simulink model "sampleModel1417_5_sub_sub_sub"  (R2023a)
settings: Solver=VariableStepAuto  StartTime=0.0  StopTime=10.0  RelTol=1e-3
libraries: hdlsllib x6, simulink x3
settings Model: Creator=user1  LastModifiedBy=user1
settings OptimizationCC: BlockReduction=off  ConditionallyExecuteInputs=off

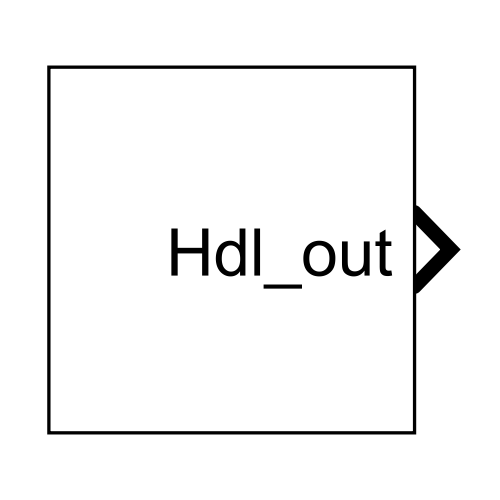
[thumbnail: Simulink's stored preview of the top-level diagram]
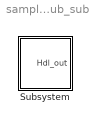
== system sampleModel1417_5_sub_sub_sub ==
  Subsystem : Subsystem

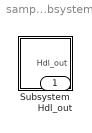
== system sampleModel1417_5_sub_sub_sub/Subsystem ==
  Subsystem : Subsystem
  Hdl_out : Outport  OutDataTypeStr=uint8

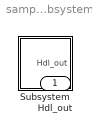
== system sampleModel1417_5_sub_sub_sub/Subsystem/Subsystem ==
  Subsystem : Subsystem
  Hdl_out : Outport  OutDataTypeStr=uint8

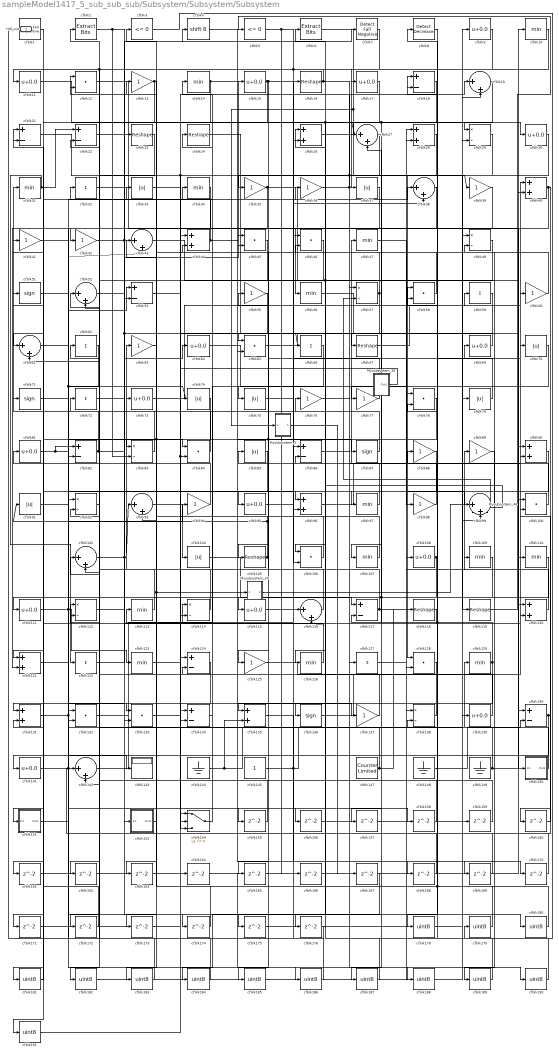
== system sampleModel1417_5_sub_sub_sub/Subsystem/Subsystem/Subsystem ==
  Mysubsystem_24 : Subsystem  TreatAsAtomicUnit=on  RTWFcnName=Mysubsystem_24
      settings: RTWFcnNameOpts=User specified  RTWFileNameOpts=Use function name
  Mysubsystem_35 : Subsystem  TreatAsAtomicUnit=on  RTWFcnName=Mysubsystem_35
      settings: RTWFcnNameOpts=User specified  RTWFileNameOpts=Use function name
  Mysubsystem_44 : Subsystem  TreatAsAtomicUnit=on  RTWFcnName=Mysubsystem_44
      settings: RTWFcnNameOpts=User specified  RTWFileNameOpts=Use function name
  Mysubsystem_5 : Subsystem  TreatAsAtomicUnit=on  RTWFcnName=Mysubsystem_5
      settings: RTWFcnNameOpts=User specified  RTWFileNameOpts=Use function name
  cfblk1 : hdlsllib/Logic and Bit Operations/Detect Fall Nonpositive  vinit=0  OutDataTypeStr=uint8
  cfblk{10,14,31,34,47,56,97,107,109..110,113,123,126,129} (14 alike) : MinMax  OutDataTypeStr=uint8
  cfblk{12,45..46,58,65,78,84,100,106,128,132..133} (12 alike) : DotProduct  OutDataTypeStr=uint8
  cfblk{19,27,38,43,52,61,93,99,102,116,142} (11 alike) : Sum  Inputs=|++  OutDataTypeStr=uint8
  cfblk{33,37,70,74..75,79,85,91,104} (9 alike) : Abs  OutDataTypeStr=uint8  SaturateOnIntegerOverflow=off
  cfblk{16,23..24,67,105,118..119} (7 alike) : Reshape
  cfblk{9,11,15,17,30,64,69,73,81,95,108,111,115,139,141} (15 alike) : Bias  Bias=0.0  SaturateOnIntegerOverflow=off
  cfblk{29,49,57,83,92,112,114,138} (8 alike) : Product  Inputs=*/  OutDataTypeStr=uint8  RndMeth=Zero  SaturateOnIntegerOverflow=on
  cfblk{18,21..22,53,82,86,117,124,134,140} (10 alike) : Sum  Inputs=+-  OutDataTypeStr=uint8
  cfblk{26,28,40,44,90,96,120..121,131,135} (10 alike) : Sum  OutDataTypeStr=uint8
  cfblk{32,59,62,66,72,122,127} (7 alike) : Sum  Inputs=+  OutDataTypeStr=uint8
  cfblk{13,35..36,39,41..42,55,60,63,76..77,88..89,94,98,125,137} (17 alike) : Gain  OutDataTypeStr=uint8
  cfblk{51,71,87,136} (4 alike) : Signum
  cfblk143 : Display
  cfblk144 : Ground
  cfblk145 : Constant  OutDataTypeStr=uint8  SampleTime=-1
  cfblk147 : hdlsllib/Sources/Counter Limited  uplimit=7  tsamp=-1
  cfblk148 : Ground
  cfblk149 : Ground
  cfblk150 : Subsystem
      settings: LibrarySourceBlock=|
      | hdlsllib/Ports &
      | Subsystems/Subsystem
  cfblk151 : Subsystem
      settings: LibrarySourceBlock=|
      | hdlsllib/Ports &
      | Subsystems/Subsystem
  cfblk153 : Subsystem
      settings: LibrarySourceBlock=|
      | hdlsllib/Ports &
      | Subsystems/Subsystem
  cfblk154 : Switch  OutDataTypeStr=uint8  SaturateOnIntegerOverflow=off  InputSameDT=off
  cfblk{155..176} (22 alike) : Delay  SampleTime=1
  cfblk{178..191} (14 alike) : DataTypeConversion  OutDataTypeStr=uint8  SaturateOnIntegerOverflow=off  RndMeth=Floor
  cfblk2 : simulink/Logic and Bit Operations/Extract Bits  bitsToExtract=Upper half  numBits=8  bitIdxRange=[0 7]  outScalingMode=Preserve fixed-point scaling
      settings: LibrarySourceBlock=|
      | hdlsllib/Logic and Bit
      | Operations/Extract Bits
  cfblk3 : hdlsllib/Logic and Bit Operations/Compare To Zero  relop=<=  OutDataTypeStr=uint8
  cfblk4 : ArithShift  BitShiftNumber=8
  cfblk5 : hdlsllib/Logic and Bit Operations/Compare To Zero  relop=<=  OutDataTypeStr=uint8
  cfblk6 : simulink/Logic and Bit Operations/Extract Bits  bitsToExtract=Upper half  numBits=8  bitIdxRange=[0 7]  outScalingMode=Preserve fixed-point scaling
      settings: LibrarySourceBlock=|
      | hdlsllib/Logic and Bit
      | Operations/Extract Bits
  cfblk7 : hdlsllib/Logic and Bit Operations/Detect Fall Negative  vinit=0  OutDataTypeStr=uint8
  cfblk8 : simulink/Logic and Bit Operations/Detect Decrease  vinit=0.0  OutDataTypeStr=uint8
      settings: LibrarySourceBlock=|
      | hdlsllib/Logic and Bit
      | Operations/Detect
      | Decrease
  Hdl_out : Outport  OutDataTypeStr=uint8
  wires:
  cfblk28/1 -> cfblk128/1
  cfblk81/1 -> cfblk53/1, cfblk82/1
  cfblk10/1 -> cfblk37/1
  cfblk69/1 -> cfblk65/1
  cfblk98/1 -> cfblk47/1
  cfblk125/1 -> cfblk40/1
  cfblk67/1 -> cfblk59/1
  cfblk114/1 -> cfblk63/1
  cfblk66/1 -> cfblk113/1
  cfblk119/1 -> cfblk5/1
  cfblk4/1 -> cfblk87/1
  cfblk84/1 -> cfblk32/1
  cfblk40/1 -> cfblk121/2, cfblk142/1
  cfblk142/1 -> cfblk114/1
  cfblk7/1 -> cfblk26/2, cfblk172/1, cfblk171/1
  cfblk16/1 -> cfblk11/1, cfblk168/1, cfblk39/1
  cfblk150/1(Out1) -> cfblk129/1
  cfblk102/1 -> cfblk45/2, cfblk93/1
  cfblk60/1 -> cfblk15/1
  cfblk65/1 -> cfblk67/1
  cfblk82/1 -> cfblk7/1, cfblk31/1
  cfblk1/1 -> cfblk61/1
  cfblk117/1 -> cfblk45/1, cfblk28/1
  cfblk87/1 -> cfblk21/1
  cfblk73/1 -> cfblk60/1
  cfblk120/1 -> cfblk89/1
  cfblk32/1 -> cfblk150/1(In1)
  cfblk12/1 -> cfblk56/1
  cfblk93/1 -> cfblk104/1
  cfblk39/1 -> cfblk96/1
  cfblk35/1 -> cfblk162/1, cfblk140/1
  cfblk139/1 -> cfblk73/1
  cfblk6/1 -> cfblk119/1, Mysubsystem_5/1(In1)
  cfblk106/1 -> cfblk71/1
  cfblk31/1 -> cfblk22/1, cfblk122/1
  cfblk26/1 -> cfblk30/1
  cfblk24/1 -> cfblk98/1
  cfblk53/1 -> cfblk44/1
  cfblk15/1 -> cfblk141/1, cfblk38/2, cfblk75/1
  cfblk148/1 -> cfblk140/2
  cfblk14/1 -> cfblk137/1, cfblk142/2
  cfblk9/1 -> cfblk17/1
  cfblk141/1 -> cfblk186/1, cfblk94/1
  cfblk21/1 -> cfblk57/1, cfblk114/2
  cfblk149/1 -> cfblk44/2, cfblk90/1
  cfblk43/1 -> cfblk100/1
  cfblk113/1 -> cfblk62/1
  cfblk104/1 -> cfblk117/1
  cfblk2/1 -> cfblk83/2, cfblk175/1, cfblk66/1
  cfblk34/1 -> cfblk132/2
  cfblk107/1 -> cfblk72/1
  cfblk116/1 -> cfblk2/1
  cfblk13/1 -> cfblk183/1, cfblk53/2
  cfblk37/1 -> cfblk83/1
  cfblk147/1 -> cfblk118/1, cfblk52/1
  cfblk96/1 -> cfblk40/2
  cfblk140/1 -> cfblk161/1, cfblk160/1
  cfblk115/1 -> cfblk16/1
  cfblk58/1 -> cfblk24/1
  cfblk56/1 -> cfblk110/1
  cfblk27/1 -> cfblk115/1
  cfblk62/1 -> cfblk82/2
  cfblk23/1 -> cfblk42/1
  cfblk132/1 -> cfblk86/1
  cfblk137/1 -> cfblk26/1
  cfblk5/1 -> cfblk166/1, cfblk78/1
  cfblk41/1 -> cfblk180/1
  cfblk74/1 -> cfblk121/1
  cfblk70/1 -> cfblk107/1
  cfblk128/1 -> cfblk124/2
  cfblk153/1(Out1) -> cfblk3/1
  cfblk49/1 -> cfblk116/2, cfblk102/2
  cfblk83/1 -> cfblk12/1
  cfblk61/1 -> cfblk84/1
  cfblk77/1 -> cfblk55/1
  cfblk78/1 -> cfblk165/1, cfblk191/1, cfblk163/1
  cfblk29/1 -> cfblk97/1
  cfblk75/1 -> cfblk70/1
  cfblk94/1 -> cfblk13/1
  cfblk17/1 -> cfblk106/1, cfblk133/1, Mysubsystem_24/1(In1)
  cfblk97/1 -> cfblk6/1
  cfblk112/1 -> cfblk120/2
  cfblk118/1 -> cfblk117/2
  cfblk127/1 -> cfblk109/1
  cfblk64/1 -> cfblk106/2
  cfblk42/1 -> cfblk4/1, cfblk153/1(In1)
  cfblk59/1 -> cfblk135/1
  cfblk111/1 -> cfblk133/2, cfblk123/1
  cfblk55/1 -> cfblk134/2
  cfblk144/1 -> cfblk135/2, cfblk9/1
  cfblk11/1 -> cfblk29/1
  cfblk72/1 -> cfblk96/2
  cfblk30/1 -> cfblk35/1
  cfblk126/1 -> cfblk51/1
  cfblk100/1 -> cfblk85/1
  cfblk47/1 -> cfblk99/1
  cfblk22/1 -> cfblk23/1
  cfblk86/1 -> cfblk90/2
  cfblk122/1 -> cfblk64/1
  cfblk63/1 -> cfblk33/1
  cfblk36/1 -> cfblk18/1, cfblk127/1
  cfblk79/1 -> cfblk58/1
  cfblk44/1 -> cfblk170/1, cfblk21/2
  cfblk131/1 -> cfblk43/2, cfblk143/1
  cfblk91/1 -> cfblk38/1
  cfblk108/1 -> cfblk18/2, cfblk187/1, cfblk136/1
  cfblk134/1 -> cfblk14/1
  cfblk129/1 -> cfblk131/1, cfblk88/1, cfblk27/2
  cfblk85/1 -> cfblk151/1(In1)
  cfblk95/1 -> cfblk69/1
  cfblk90/1 -> cfblk111/1
  cfblk124/1 -> cfblk154/2
  cfblk138/1 -> cfblk112/1
  cfblk105/1 -> cfblk125/1, cfblk81/1, cfblk91/1
  cfblk154/1 -> cfblk34/1
  cfblk151/1(Out1) -> cfblk138/2
  cfblk136/1 -> cfblk10/1
  cfblk123/1 -> cfblk19/1
  cfblk133/1 -> cfblk36/1
  cfblk19/1 -> cfblk105/1
  cfblk51/1 -> cfblk95/1, cfblk74/1
  cfblk18/1 -> cfblk77/1, cfblk27/1
  cfblk99/1 -> cfblk49/2
  cfblk145/1 -> cfblk29/2, cfblk116/1
  cfblk45/1 -> cfblk52/2
  cfblk57/1 -> cfblk12/2, cfblk65/2
  cfblk33/1 -> cfblk155/1
  cfblk155/1 -> cfblk102/1
  cfblk121/1 -> cfblk156/1
  cfblk156/1 -> cfblk128/2
  cfblk38/1 -> cfblk157/1
  cfblk157/1 -> cfblk19/2
  cfblk71/1 -> cfblk158/1
  cfblk158/1 -> cfblk61/2
  cfblk159/1 -> cfblk93/2
  cfblk160/1 -> cfblk100/2
  cfblk161/1 -> cfblk99/2
  cfblk162/1 -> cfblk22/2
  cfblk163/1 -> cfblk120/1
  cfblk165/1 -> cfblk28/2
  cfblk166/1 -> cfblk138/1
  cfblk168/1 -> cfblk112/2
  cfblk135/1 -> cfblk169/1
  cfblk169/1 -> cfblk132/1
  cfblk170/1 -> cfblk86/2
  cfblk171/1 -> cfblk124/1
  cfblk172/1 -> cfblk131/2
  cfblk109/1 -> cfblk173/1
  cfblk173/1 -> cfblk154/1
  cfblk52/1 -> cfblk174/1
  cfblk174/1 -> cfblk43/1
  cfblk175/1 -> cfblk49/1
  cfblk88/1 -> cfblk176/1
  cfblk176/1 -> cfblk1/1
  cfblk8/1 -> cfblk178/1
  cfblk178/1 -> cfblk139/1
  cfblk3/1 -> cfblk179/1
  cfblk179/1 -> cfblk8/1
  cfblk180/1 -> cfblk134/1, cfblk78/2
  cfblk110/1 -> cfblk181/1
  cfblk181/1 -> cfblk41/1
  cfblk92/1 -> cfblk182/1
  cfblk182/1 -> cfblk108/1
  cfblk183/1 -> cfblk92/1
  cfblk167/1 -> cfblk184/1
  cfblk184/1 -> cfblk92/2
  cfblk46/1 -> cfblk185/1
  cfblk185/1 -> cfblk159/1
  cfblk186/1 -> cfblk46/1
  cfblk187/1 -> cfblk46/2
  cfblk76/1 -> cfblk188/1
  cfblk188/1 -> cfblk79/1
  cfblk89/1 -> cfblk189/1
  cfblk189/1 -> cfblk76/1
  cfblk164/1 -> cfblk190/1
  cfblk190/1 -> cfblk58/2
  cfblk191/1 -> cfblk164/1
  Mysubsystem_5/1(Out1) -> cfblk167/1
  Mysubsystem_35/1(Out1) -> cfblk154/3, cfblk84/2
  Mysubsystem_24/1(Out1) -> Mysubsystem_44/1(In1)
  Mysubsystem_44/1(Out1) -> cfblk57/2
  Mysubsystem_44/2(Out2) -> cfblk126/1

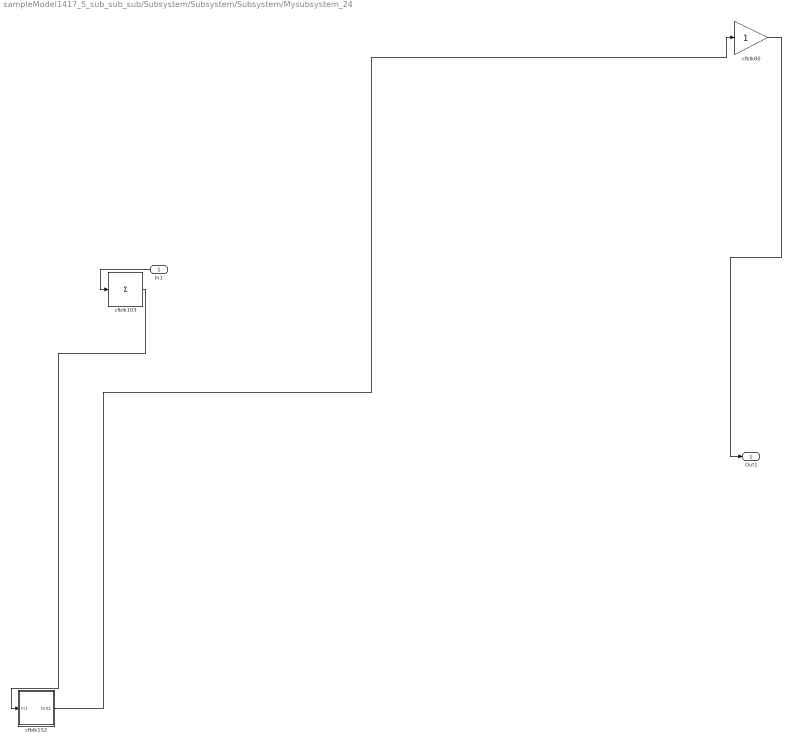
== system sampleModel1417_5_sub_sub_sub/Subsystem/Subsystem/Subsystem/Mysubsystem_24 ==
  In1 : Inport
  cfblk103 : Sum  Inputs=+
  cfblk152 : Subsystem
      settings: LibrarySourceBlock=|
      | hdlsllib/Ports &
      | Subsystems/Subsystem
  cfblk80 : Gain
  Out1 : Outport
  wires:
  In1/1 -> cfblk103/1
  cfblk80/1 -> Out1/1
  cfblk103/1 -> cfblk152/1(In1)
  cfblk152/1(Out1) -> cfblk80/1

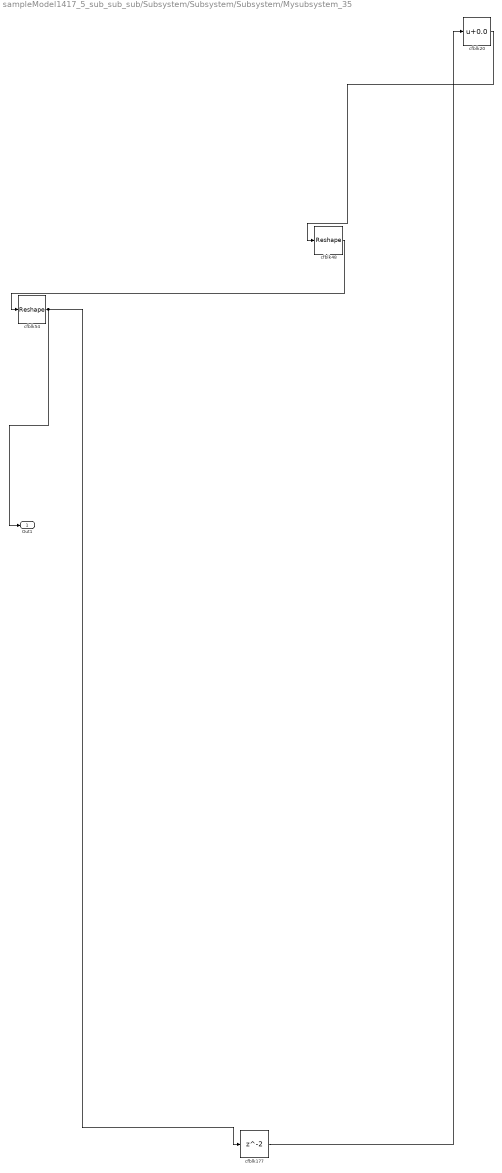
== system sampleModel1417_5_sub_sub_sub/Subsystem/Subsystem/Subsystem/Mysubsystem_35 ==
  cfblk177 : Delay  SampleTime=1
  cfblk20 : Bias  Bias=0.0  SaturateOnIntegerOverflow=off
  cfblk48 : Reshape
  cfblk54 : Reshape
  Out1 : Outport
  wires:
  cfblk20/1 -> cfblk48/1
  cfblk48/1 -> cfblk54/1
  cfblk177/1 -> cfblk20/1
  cfblk54/1 -> cfblk177/1, Out1/1

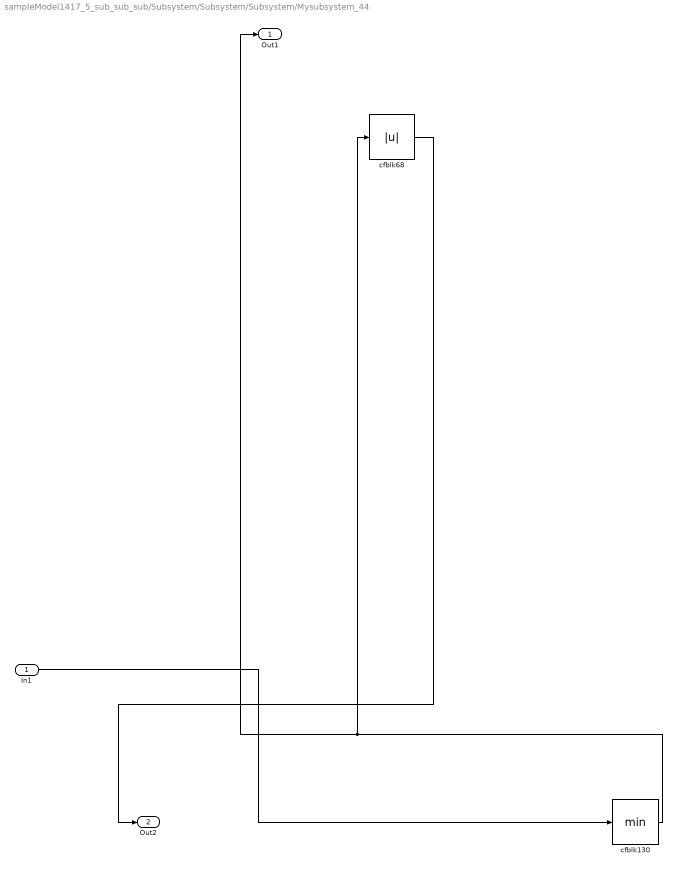
== system sampleModel1417_5_sub_sub_sub/Subsystem/Subsystem/Subsystem/Mysubsystem_44 ==
  In1 : Inport
  cfblk130 : MinMax
  cfblk68 : Abs  SaturateOnIntegerOverflow=off
  Out1 : Outport
  Out2 : Outport  Port=2
  wires:
  cfblk68/1 -> Out2/1
  In1/1 -> cfblk130/1
  cfblk130/1 -> cfblk68/1, Out1/1

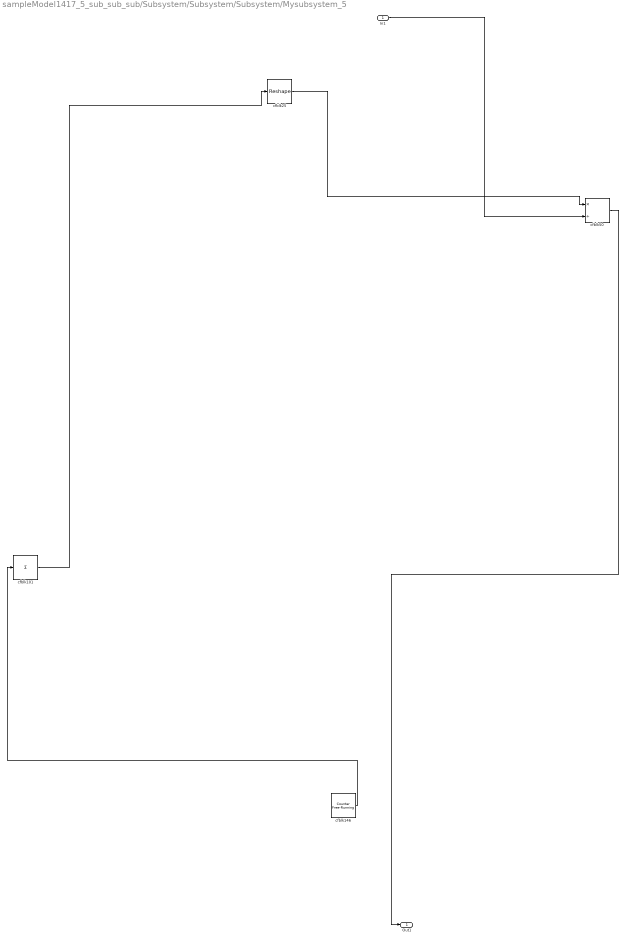
== system sampleModel1417_5_sub_sub_sub/Subsystem/Subsystem/Subsystem/Mysubsystem_5 ==
  In1 : Inport
  cfblk101 : Sum  Inputs=+
  cfblk146 : hdlsllib/Sources/Counter Free-Running  NumBits=16  tsamp=-1
  cfblk25 : Reshape
  cfblk50 : Product  Inputs=*/  RndMeth=Zero  SaturateOnIntegerOverflow=on
  Out1 : Outport
  wires:
  cfblk101/1 -> cfblk25/1
  In1/1 -> cfblk50/2
  cfblk50/1 -> Out1/1
  cfblk146/1 -> cfblk101/1
  cfblk25/1 -> cfblk50/1

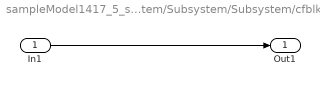
== system sampleModel1417_5_sub_sub_sub/Subsystem/Subsystem/Subsystem/cfblk150 ==
  In1 : Inport
  Out1 : Outport
  wires:
  In1/1 -> Out1/1

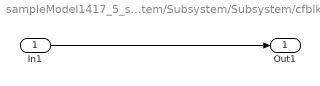
== system sampleModel1417_5_sub_sub_sub/Subsystem/Subsystem/Subsystem/cfblk151 ==
  In1 : Inport
  Out1 : Outport
  wires:
  In1/1 -> Out1/1

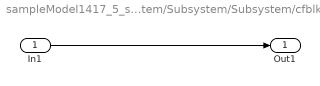
== system sampleModel1417_5_sub_sub_sub/Subsystem/Subsystem/Subsystem/cfblk153 ==
  In1 : Inport
  Out1 : Outport
  wires:
  In1/1 -> Out1/1

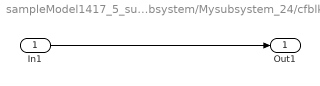
== system sampleModel1417_5_sub_sub_sub/Subsystem/Subsystem/Subsystem/Mysubsystem_24/cfblk152 ==
  In1 : Inport
  Out1 : Outport
  wires:
  In1/1 -> Out1/1
